simulink model "Model"  (R2019b)
settings: Solver=VariableStepAuto  StartTime=0.0  StopTime=4  MaxStep=1e-3  RelTol=1e-3
values from neighbouring files (symbols this model uses):
  fsin = 1    [SinTr.m]
  ftr = 8    [SinTr.m]
  k = 8    [SinTr.m]
libraries: simulink x1
settings Model: Creator=atmat  LastModifiedBy=atmat

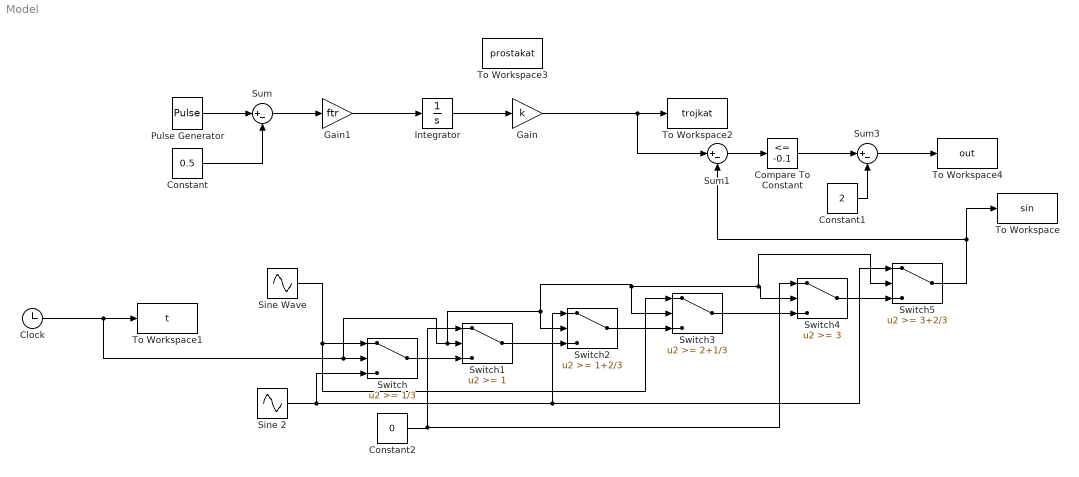
== system Model ==
  Clock : Clock
  Compare To Constant : simulink/Logic and Bit Operations/Compare To Constant  relop=<=  const=-0.1  OutDataTypeStr=boolean
  Constant : Constant  Value=0.5
  Constant1 : Constant  Value=2
  Constant2 : Constant  Value=0
  Gain : Gain  Gain=k
  Gain1 : Gain  Gain=ftr
  Integrator : Integrator
  Pulse Generator : DiscretePulseGenerator  PulseType=Time based  Period=1/ftr  PulseWidth=50
  "Sine 2 " : Sin  Frequency=fsin*(pi)  Phase=fsin*(pi)/3  SampleTime=0
  Sine Wave : Sin  Frequency=fsin*(pi)  SampleTime=0
  Sum : Sum  Inputs=|+-
  Sum1 : Sum  Inputs=|+-
  Sum3 : Sum  Inputs=|+-
  Switch : Switch  Threshold=1/3
  Switch1 : Switch  Threshold=1
  Switch2 : Switch  Threshold=1+2/3
  Switch3 : Switch  Threshold=2+1/3
  Switch4 : Switch  Threshold=3
  Switch5 : Switch  Threshold=3+2/3
  To Workspace : ToWorkspace  VariableName=sin  SampleTime=-1
  To Workspace1 : ToWorkspace  VariableName=t  SampleTime=-1
  To Workspace2 : ToWorkspace  VariableName=trojkat  SampleTime=-1
  To Workspace3 : ToWorkspace  VariableName=prostakat  SampleTime=-1
  To Workspace4 : ToWorkspace  VariableName=out  SampleTime=-1
  wires:
  Pulse Generator/1 -> Sum/1
  Constant/1 -> Sum/2
  Integrator/1 -> Gain/1
  Sum1/1 -> Compare To Constant/1
  Gain/1 -> Sum1/1, To Workspace2/1
  Gain1/1 -> Integrator/1
  Sum/1 -> Gain1/1
  Sine Wave/1 -> Switch3/1, Switch/1
  Clock/1 -> Switch2/2, Switch5/2, Switch4/2, Switch3/2, Switch1/2, Switch/2, To Workspace1/1
  Switch/1 -> Switch1/3
  Constant2/1 -> Switch4/1, Switch1/1
  Switch1/1 -> Switch2/3
  Switch2/1 -> Switch3/3
  Switch3/1 -> Switch4/3
  Switch4/1 -> Switch5/3
  "Sine 2 "/1 -> Switch5/1, Switch2/1, Switch/3
  Switch5/1 -> To Workspace/1, Sum1/2
  Sum3/1 -> To Workspace4/1
  Compare To Constant/1 -> Sum3/1
  Constant1/1 -> Sum3/2
